simulink model "simu_2"  (R2019b)
settings: Solver=VariableStepAuto  StartTime=0.0  StopTime=2.5  RelTol=1e-3
settings Model: Creator=Romain  LastModifiedBy=Romain

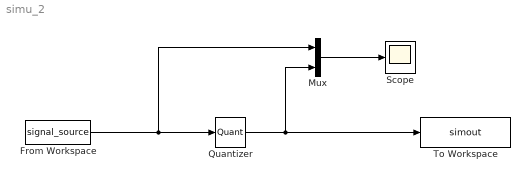
== system simu_2 ==
  From Workspace : FromWorkspace  VariableName=signal_source  SampleTime=0
  Mux : Mux  Inputs=2
  Quantizer : Quantizer
  Scope : Scope
  To Workspace : ToWorkspace  VariableName=simout  SaveFormat=Timeseries  SampleTime=-1
  wires:
  From Workspace/1 -> Mux/1, Quantizer/1
  Quantizer/1 -> Mux/2, To Workspace/1
  Mux/1 -> Scope/1
